simulink model "controlled_full_RL_high"  (R2022b)
settings: Solver=VariableStepAuto  StartTime=0.0  StopTime=00.04  RelTol=1e-3
libraries: spsThyristorLib x4, spsCurrentMeasurementLib x3, spsVoltageMeasurementLib x3, spsACVoltageSourceLib x1, spsSeriesRLCBranchLib x1, sps_lib x1
settings Model: Creator=mroun  LastModifiedBy=mroun

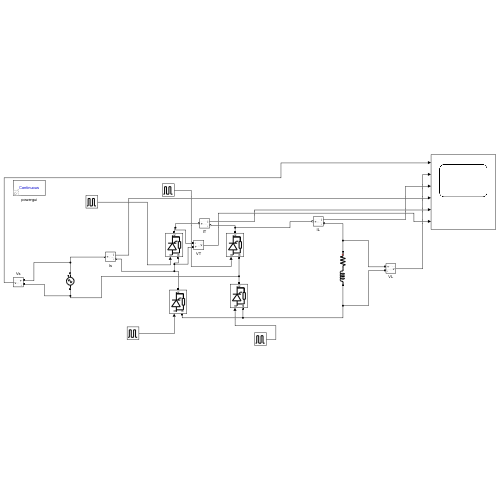
[thumbnail: Simulink's stored preview of the top-level diagram]
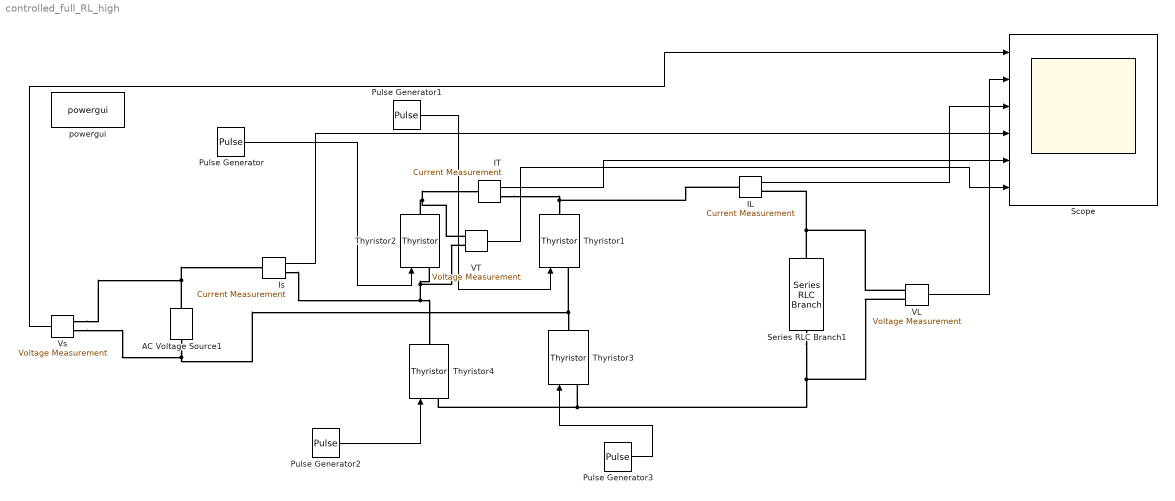
== system controlled_full_RL_high ==
  AC Voltage Source1 : spsACVoltageSourceLib/AC Voltage Source  Amplitude=200  Phase=0  Frequency=50  SampleTime=0  Measurements=None  BusType=swing  Pref=10e3  Qref=0  Qmin=-inf  Qmax=+inf
  IL : spsCurrentMeasurementLib/Current Measurement  PhasorSimulation=off  OutputType=Complex  PSBequivalent=0
  IT : spsCurrentMeasurementLib/Current Measurement  PhasorSimulation=off  OutputType=Complex  PSBequivalent=0
  Is : spsCurrentMeasurementLib/Current Measurement  PhasorSimulation=off  OutputType=Complex  PSBequivalent=0
  Pulse Generator : DiscretePulseGenerator  PulseType=Time based  Period=.02  PulseWidth=5  PhaseDelay=(30)/(180*100)
  Pulse Generator1 : DiscretePulseGenerator  PulseType=Time based  Period=.02  PulseWidth=5  PhaseDelay=(30+180)/(180*100)
  Pulse Generator2 : DiscretePulseGenerator  PulseType=Time based  Period=.02  PulseWidth=5  PhaseDelay=(30+180)/(180*100)
  Pulse Generator3 : DiscretePulseGenerator  PulseType=Time based  Period=.02  PulseWidth=5  PhaseDelay=(30)/(180*100)
  Scope : Scope  NumInputPorts=6
  Series RLC Branch1 : spsSeriesRLCBranchLib/Series RLC Branch  LConnTagsString=__new0  RConnTagsString=__new0  BranchType=RL  Resistance=10  Inductance=.025  SetiL0=off  InitialCurrent=.1  Capacitance=1e-6  Setx0=off  InitialVoltage=0  Measurements=None
  Thyristor{1..4} (4 alike) : spsThyristorLib/Thyristor  Ron=0.001  Lon=0  Vf=0.8  IC=0  Rs=500  Cs=250e-9  Measurements=off
  VL : spsVoltageMeasurementLib/Voltage Measurement  PhasorSimulation=off  OutputType=Complex  PSBequivalent=0
  VT : spsVoltageMeasurementLib/Voltage Measurement  PhasorSimulation=off  OutputType=Complex  PSBequivalent=0
  Vs : spsVoltageMeasurementLib/Voltage Measurement  PhasorSimulation=off  OutputType=Complex  PSBequivalent=0
  powergui : sps_lib/powergui  Priority=1  SimulationMode=Continuous  SampleTime=50e-6  frequency=60  Iterations=50  frequencyindice=50  Pbase=100e6  ErrMax=1e-4  UnitsV=kV  UnitsW=MW  buscounter=0  FunctionMessages=off  echomessages=off  EnableUseOfTLC=off  CurrentSourceSwitches=off  DisableSnubberDevices=off  DisableRonSwitches=off  DisableVfSwitches=off  DisplayEquations=off  AutomaticDiscreteSolvers=off  SolverType=Tustin/Backward Euler (TBE)  Interpol=off  ExternalGateDelay=off  methode=off  Ts=100  x0status=blocks  SPID=on  SwTol=0  HookPort=off  NonlinearTolerance=1e-4  nMaxIteration=100  ContinueOnMaxIteration=off  RestoreLinks=warning  ResistiveCurrentMeasurement=off  Frange=[0:2:500]  Ylog=off  Xlog=on  ShowGrid=off  save=off  variable=ZData  structure=0  ZoomFFT=off  StartTime=0.0  cycles=1  DisplayStyle=1  fundamental=60  FreqAxis=off  MaxFrequency=1000  frequencyindicesteady=1  RmsSteady=1  display=off
  wires:
  Vs/1 -> Scope/1
  VL/1 -> Scope/2
  IL/1 -> Scope/3
  Is/1 -> Scope/4
  IT/1 -> Scope/5
  VT/1 -> Scope/6
  Pulse Generator/1 -> Thyristor2/1
  Pulse Generator1/1 -> Thyristor1/1
  Pulse Generator2/1 -> Thyristor4/1
  Pulse Generator3/1 -> Thyristor3/1
  connections:
  Thyristor1/RConn1 -- IL/LConn1 -- IT/RConn1
  VT/LConn1 -- Is/RConn1 -- Thyristor4/RConn1 -- Thyristor2/LConn1
  Vs/LConn2 -- AC Voltage Source1/LConn1 -- Thyristor3/RConn1 -- Thyristor1/LConn1
  VL/LConn2 -- Series RLC Branch1/RConn1 -- Thyristor4/LConn1 -- Thyristor3/LConn1
  VL/LConn1 -- IL/RConn1 -- Series RLC Branch1/LConn1
  Vs/LConn1 -- AC Voltage Source1/RConn1 -- Is/LConn1
  VT/LConn2 -- IT/LConn1 -- Thyristor2/RConn1
